simulink model "SimulinkOnramp"  (R2021a)
settings: Solver=VariableStepAuto  StartTime=0.0  StopTime=10.0  RelTol=1e-3
StartFcn:
  | learning.simulink.modelCallbacks.startFunction(gcs)
StopFcn:
  | learning.simulink.modelCallbacks.stopFunction(gcs)
model workspace (MAT data in the model file):
  courseObject.course = 'simulink'
  courseObject.chapter = 10
  courseObject.lesson = 1
  courseObject.section = 1
  courseObject.task = 1
  t_ans = [0; 3.15544362088e-30; 8.93115175648e-07; 5.35869105389e-06; 2.76865704451e-05; 0.000139325967401; 0.000697522952181; 0.00348850787608; 0.0174434324956; 0.0872180555931; 0.187218055593; 0.287218055593; 0.387218055593; 0.487218055593; 0.587218055593; 0.687218055593; 0.787218055593; 0.887218055593; 0.987218055593; 1.08721805559; 1.18721805559; 1.28721805559; 1.38721805559; 1.48721805559; 1.58721805559; 1.68721805559; 1.78721805559; 1.88721805559; 1.98721805559; 2.08721805559; 2.18721805559; 2.28721805559; 2.38721805559; 2.48721805559; 2.58721805559; 2.68721805559; 2.78721805559; 2.88721805559; 2.98721805559; 3.08721805559; 3.18721805559; 3.28721805559; 3.38721805559; 3.48721805559; 3.58721805559; 3.68721805559; 3.78721805559; 3.88721805559; 3.98721805559; 4.08721805559; 4.18721805559; 4.28721805559; 4.38721805559; 4.48721805559; 4.58721805559; 4.68721805559; 4.78721805559; 4.88721805559; 4.98721805559; 5.08721805559; 5.18721805559; 5.28721805559; 5.38721805559; 5.48721805559; 5.58721805559; 5.68721805559; 5.78721805559; 5.88721805559; 5.98721805559; 6.08721805559; 6.18721805559; 6.28721805559; 6.38721805559; 6.48721805559; 6.58721805559; 6.68721805559; 6.78721805559; 6.88721805559; 6.98721805559; 7.08721805559; 7.18721805559; 7.28721805559; 7.38721805559; 7.48721805559; 7.58721805559; 7.68721805559; 7.78721805559; 7.88721805559; 7.98721805559; 8.08721805559; 8.18721805559; 8.28721805559; 8.38721805559; 8.48721805559; 8.58721805559; 8.68721805559; 8.78721805559; 8.88721805559; 8.98721805559; 9.08721805559; 9.18721805559; 9.28721805559; 9.38721805559; 9.48721805559; 9.58721805559; 9.68721805559; 9.78721805559; 9.88721805559; 9.98721805559; 10]
  y_ans5 = [0; 7.09974814699e-28; 0.000200950847219; 0.00120570306425; 0.00622941367326; 0.031346704858; 0.156901619732; 0.78388834969; 3.89921084005; 18.9959918903; 39.3003618294; 58.1376087854; 75.6137419502; 91.827110661; 106.868957875; 120.82393365; 133.770571529; 145.781730491; 156.925004982; 167.263105308; 176.854210547; 185.75229596; 194.007436743; 201.666089834; 208.771355353; 215.363219157; 221.478777865; 227.152447622; 232.416157782; 237.299530598; 241.830047919; 246.033205854; 249.93265825; 253.550349811; 256.906639593; 260.020415576; 262.909200962; 265.589252788; 268.075653413; 270.382395397; 272.522460247; 274.507891472; 276.349862359; 278.058738852; 279.644137887; 281.114981515; 282.47954711; 283.745513953; 284.920006446; 286.009634205; 287.020529262; 287.958380566; 288.828466005; 289.635682103; 290.38457158; 291.079348915; 291.723924061; 292.321924455; 292.876715425; 293.391419134; 293.868932148; 294.311941735; 294.722940995; 295.104242881; 295.457993222; 295.786182796; 296.090658536; 296.373133921; 296.635198619; 296.878327436; 297.103888612; 297.313151524; 297.507293828; 297.687408085; 297.854507914; 298.009533692; 298.153357848; 298.286789772; 298.41058037; 298.525426291; 298.631973847; 298.730822647; 298.822528978; 298.907608929; 298.986541299; 299.059770291; 299.127708012; 299.19073679; 299.249211328; 299.3034607; 299.353790202; 299.400483069; 299.443802072; 299.483990995; 299.521276007; 299.555866934; 299.587958441; 299.617731127; 299.645352543; 299.670978132; 299.694752105; 299.716808254; 299.737270702; 299.756254605; 299.773866797; 299.790206394; 299.805365349; 299.81942897; 299.832476403; 299.834074688]
  y_ans6 = [320; 320; 319.999986603; 319.99991962; 319.999584706; 319.99791022; 319.989539892; 319.947740777; 319.740052611; 318.733600541; 317.379975878; 316.124159414; 314.95908387; 313.878192623; 312.875402808; 311.94507109; 311.081961898; 310.281217967; 309.538333001; 308.849126313; 308.209719297; 307.616513603; 307.066170884; 306.555594011; 306.081909643; 305.642452056; 305.234748142; 304.856503492; 304.505589481; 304.180031293; 303.877996805; 303.597786276; 303.337822783; 303.096643346; 302.872890694; 302.665305628; 302.472719936; 302.294049814; 302.128289772; 301.974506974; 301.831835984; 301.699473902; 301.576675843; 301.462750743; 301.357057474; 301.259001232; 301.168030193; 301.083632403; 301.005332904; 300.932691053; 300.865298049; 300.802774629; 300.744768933; 300.690954526; 300.641028561; 300.594710072; 300.551738396; 300.511871703; 300.474885638; 300.440572058; 300.408737857; 300.379203884; 300.351803934; 300.326383808; 300.302800452; 300.280921147; 300.260622764; 300.241791072; 300.224320092; 300.208111504; 300.193074093; 300.179123232; 300.166180411; 300.154172794; 300.143032806; 300.132697754; 300.123109477; 300.114214015; 300.105961309; 300.098304914; 300.091201744; 300.084611824; 300.078498068; 300.072826071; 300.067563913; 300.062681981; 300.058152799; 300.053950881; 300.050052578; 300.046435953; 300.043080653; 300.039967795; 300.037079862; 300.0344006; 300.031914933; 300.029608871; 300.027469437; 300.025484592; 300.023643164; 300.021934791; 300.02034986; 300.01887945; 300.017515287; 300.016249693; 300.015075547; 300.01398624; 300.012975643; 300.012038069; 300.01116824; 300.011061687]
undefined symbols (not defined in the file): r
libraries: signalChecks x1
CloseFcn:
  | learning.simulink.cleanupOnlineTraining
settings Model: Creator=HP  LastModifiedBy=HP
settings DataIOCC: SaveTime=off

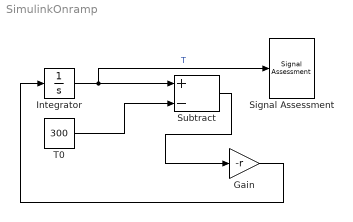
== system SimulinkOnramp ==
  Gain : Gain  Gain=-r
  Integrator : Integrator  InitialCondition=320
  Signal Assessment : signalChecks/Signal Assessment  signal_type='signal'  t_ans=t_ans  y_ans_upper=y_ans6  y_ans_lower=0  range=.01  rate_type=0  lesson=0  task=6  pass=1
  Subtract : Sum  Inputs=+-
  T0 : Constant  Value=300
  wires:
  Integrator/1 -> Signal Assessment/1, Subtract/1  "T"
  T0/1 -> Subtract/2
  Subtract/1 -> Gain/1
  Gain/1 -> Integrator/1
